simulink model "NanoBalancerCascade"  (R2022b)
settings: Solver=FixedStepAuto  StartTime=0.0  StopTime=inf  RelTol=1e-3  EnableMultiTasking=on
model workspace (MAT data in the model file):
  Saturation = 0.85
  sampleTime = 0.01
libraries: arduinomotorcarrierlib x5, simulink_extras x3, slpidlib x2, simulink x2, eeGeneralControl x2, arduinosensorlib x1, arduinolib x1
settings Model: ExtModeTrigDuration=2  Creator=arkad  LastModifiedBy=arkad
settings OptimizationCC: EnhancedBackFolding=on  PassReuseOutputArgsAs=Individual arguments  ZeroExternalMemoryAtStartup=off  ZeroInternalMemoryAtStartup=off  MaxStackSize=64  OptimizeBlockOrder=speed  DifferentSizesBufferReuse=on  OptimizationCustomize=off  EfficientTunableParamExpr=on
settings DebuggingCC: ParameterTunabilityLossMsg=error
settings HardwareCC: ProdBitPerPointer=32  ProdBitPerSizeT=32  ProdBitPerPtrDiffT=32  ProdLargestAtomicInteger=Long  ProdLargestAtomicFloat=Double  ProdWordSize=32  ProdHWDeviceType=ARM Compatible->ARM Cortex
settings SFSimCC: MATLABDynamicMemAlloc=off
settings RTWCC: Description=Embedded Coder  SystemTargetFile=ert.tlc  HardwareBoard=Arduino Nano 33 IoT  TLCOptions=-aInlineSetEventsForThisBaseRateFcn=TLC_FALSE -aSuppressMultiTaskScheduler=TLC_FALSE -aRateBasedStepFcn=1  TemplateMakefile=ert_default_tmf  Toolchain=Arduino ARM  BuildConfiguration=Faster Runs
settings CodeAppCC: ForceParamTrailComments=on  IgnoreCustomStorageClasses=off  OperatorAnnotations=on  SimulinkDataObjDesc=on  SFDataObjDesc=on  InsertBlockDesc=on
settings ERTTargetCC: SupportContinuousTime=on  SupportVariableSizeSignals=on  ExtModeTransport=2  ExtModeStaticAlloc=on  ExtModeAutomaticAllocSize=off  ExtModeStaticAllocSize=8192  ExtModeMexFile=ext_xcp  ExtModeIntrfLevel=Level2 - Open

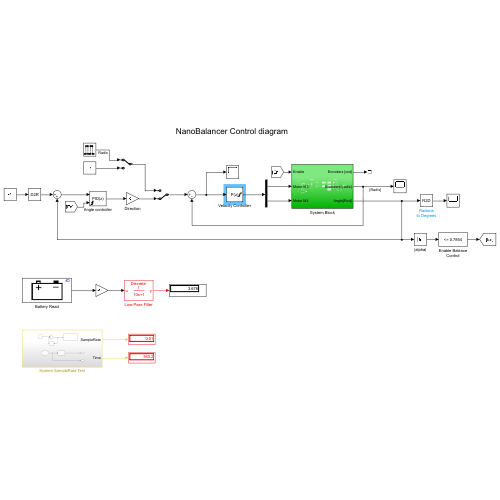
[thumbnail: Simulink's stored preview of the top-level diagram]
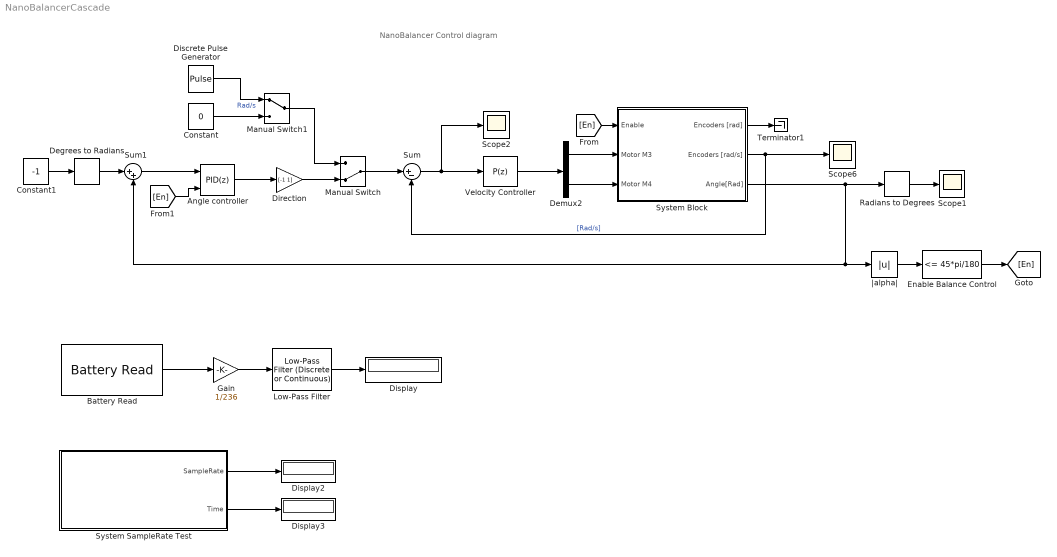
== system NanoBalancerCascade ==
  note: NanoBalancer Control diagram
  Angle controller : slpidlib/PID Controller  Controller=PID  Form=Parallel  TimeDomain=Discrete-time  UseExternalTs=off  SampleTime=-1  IntegratorMethod=Forward Euler  FilterMethod=Forward Euler  ControllerParametersSource=internal  P=175  I=10  UseKiTs=on  D=10  N=30  UseFilter=on  TunerSelectOption=Transfer Function Based (PID Tuner App)  InitialConditionSource=internal  InitialConditionForIntegrator=0  InitialConditionForFilter=0  DifferentiatorICPrevScaledInput=0  ExternalReset=rising  TrackingMode=off  Kt=1  LimitOutput=off  SatLimitsSource=internal  UpperSaturationLimit=100  LowerSaturationLimit=-100  LinearizeAsGain=on  AntiWindupMode=clamping  Kb=1  LimitIntegrator=on  UpperIntegratorSaturationLimit=50  LowerIntegratorSaturationLimit=-50  POutMin=[]  POutMax=[]  IOutMin=[]  IOutMax=[]  DOutMin=[]  DOutMax=[]  NOutMin=[]  NOutMax=[]  SumOutMin=[]  SumOutMax=[]  SaturationOutMin=[]  SaturationOutMax=[]  PParamMin=[]  PParamMax=[]  IParamMin=[]  IParamMax=[]  DParamMin=[]  DParamMax=[]  NParamMin=[]  NParamMax=[]  KbParamMin=[]  KbParamMax=[]  KtParamMin=[]  KtParamMax=[]  KbOutMin=[]  KbOutMax=[]  KtOutMin=[]  KtOutMax=[]  IntegratorOutMin=[]  IntegratorOutMax=[]  FilterOutMin=[]  FilterOutMax=[]  SumI1OutMin=[]  SumI1OutMax=[]  SumI2OutMin=[]  SumI2OutMax=[]  SumI3OutMin=[]  SumI3OutMax=[]  SumI4OutMin=[]  SumI4OutMax=[]  SumDOutMin=[]  SumDOutMax=[]  DifferentiatorOutMin=[]  DifferentiatorOutMax=[]  FilterDiffOutCoefMin=[]  FilterDiffOutCoefMax=[]  ReciprocalOutMin=[]  ReciprocalOutMax=[]  SumDenOutMin=[]  SumDenOutMax=[]  SumNumOutMin=[]  SumNumOutMax=[]  DivideOutMin=[]  DivideOutMax=[]  UdiffTsProdOutMin=[]  UdiffTsProdOutMax=[]  NTsProdOutMin=[]  NTsProdOutMax=[]  UintegralTsProdOutMin=[]  UintegralTsProdOutMax=[]  UngainTsProdOutMin=[]  UngainTsProdOutMax=[]  ClampingZeroOutDataTypeStr=Inherit: Inherit via back propagation  ClampingZeroOutMin=[]  ClampingZeroOutMax=[]  FilterDenConstantOutDataTypeStr=Inherit: Inherit via back propagation  FilterDenConstantOutMin=[]  FilterDenConstantOutMax=[]  PCopyOutDataTypeStr=Inherit: Inherit via back propagation  PCopyOutMin=[]  PCopyOutMax=[]  NCopyOutDataTypeStr=Inherit: Inherit via back propagation  NCopyOutMin=[]  NCopyOutMax=[]  IntegratorContinuousStateAttributes=''  IntegratorStateMustResolveToSignalObject=off  IntegratorRTWStateStorageClass=Auto  FilterContinuousStateAttributes=''  FilterStateMustResolveToSignalObject=off  FilterRTWStateStorageClass=Auto  ParallelPVariant=InternalParameters  IdealPVariant=Disabled  IVariant=InternalParameters  DVariant=InternalParameters  IntegratorVariant=Discrete  SatVariant=Disabled  AWVariant=Passthrough  PCopyVariant=Disabled  TRVariant=Disabled  FdbkBlocksVariant=Forward  IdealPFdbkVariant=Disabled  SatFdbkVariant=Disabled  DerivativeFilterVariant=ForwardEulerFilter  NVariant=InternalParameters  NCopyVariant=Disabled  FilterICVariant=InternalICsFilter  IntegratorICVariant=InternalICs  ExternalResetVariant=ExternalReset  TRSumVariant=Passthrough  SumFdbkVariant=Disabled  SumVariant=Sum_PID  TsampFilterVariant=InternalTs  TsampNgainVariant=Passthrough  TsampIntegralVariant=Passthrough  ExternalSaturationOutDataTypeStr=Inherit: Same as second input
  Battery Read : arduinomotorcarrierlib/Battery Read  SlaveAddress=uint8( hex2dec( '66' ) )  blockPlatform=ARDUINO  SampleTime=0.1
  Constant : Constant  Value=0
  Constant1 : Constant  Value=-1
  Degrees to Radians : simulink_extras/Transformations/Degrees to Radians
  Demux2 : Demux  Outputs=2
  Direction : Gain  Gain=[-1 1]  ParamDataTypeStr=double  OutDataTypeStr=double
  Discrete Pulse Generator : DiscretePulseGenerator  Amplitude=40  Period=4/sampleTime  PulseWidth=2/sampleTime  SampleTime=sampleTime
  Display : Display
  Display2 : Display
  Display3 : Display
  Enable Balance Control : simulink/Logic and Bit Operations/Compare To Constant  relop=<=  const=45*pi/180  OutDataTypeStr=uint8  ZeroCross=off
  Gain : Gain  Gain=1/236  ParamDataTypeStr=double  OutDataTypeStr=double
  Low-Pass Filter : eeGeneralControl/Low-Pass Filter (Discrete or Continuous)  K=1  T=10  B=inf  A=-inf  init_option=Inherited from block input  x0=0  Ts=-1
  Manual Switch : ManualSwitch  CurrentSetting=0
  Manual Switch1 : ManualSwitch
  Radians to Degrees : simulink_extras/Transformations/Radians to Degrees
  Scope1 : Scope
  Scope2 : Scope
  Scope6 : Scope
  Sum : Sum  Inputs=|+-
  Sum1 : Sum  Inputs=|++
  System Block : Subsystem
  System SampleRate Test : Subsystem
  Terminator1 : Terminator
  Velocity Controller : slpidlib/PID Controller  Controller=P  Form=Parallel  TimeDomain=Discrete-time  UseExternalTs=off  SampleTime=-1  IntegratorMethod=Forward Euler  FilterMethod=Forward Euler  ControllerParametersSource=internal  P=0.01  I=0.001*0  UseKiTs=on  D=0.01  N=20  UseFilter=on  TunerSelectOption=Transfer Function Based (PID Tuner App)  InitialConditionSource=internal  InitialConditionForIntegrator=0  InitialConditionForFilter=0  DifferentiatorICPrevScaledInput=0  ExternalReset=rising  TrackingMode=off  Kt=1  LimitOutput=on  SatLimitsSource=internal  UpperSaturationLimit=1  LowerSaturationLimit=-1  LinearizeAsGain=on  AntiWindupMode=clamping  Kb=1  LimitIntegrator=off  UpperIntegratorSaturationLimit=inf  LowerIntegratorSaturationLimit=-inf  POutMin=[]  POutMax=[]  IOutMin=[]  IOutMax=[]  DOutMin=[]  DOutMax=[]  NOutMin=[]  NOutMax=[]  SumOutMin=[]  SumOutMax=[]  SaturationOutMin=[]  SaturationOutMax=[]  PParamMin=[]  PParamMax=[]  IParamMin=[]  IParamMax=[]  DParamMin=[]  DParamMax=[]  NParamMin=[]  NParamMax=[]  KbParamMin=[]  KbParamMax=[]  KtParamMin=[]  KtParamMax=[]  KbOutMin=[]  KbOutMax=[]  KtOutMin=[]  KtOutMax=[]  IntegratorOutMin=[]  IntegratorOutMax=[]  FilterOutMin=[]  FilterOutMax=[]  SumI1OutMin=[]  SumI1OutMax=[]  SumI2OutMin=[]  SumI2OutMax=[]  SumI3OutMin=[]  SumI3OutMax=[]  SumI4OutMin=[]  SumI4OutMax=[]  SumDOutMin=[]  SumDOutMax=[]  DifferentiatorOutMin=[]  DifferentiatorOutMax=[]  FilterDiffOutCoefMin=[]  FilterDiffOutCoefMax=[]  ReciprocalOutMin=[]  ReciprocalOutMax=[]  SumDenOutMin=[]  SumDenOutMax=[]  SumNumOutMin=[]  SumNumOutMax=[]  DivideOutMin=[]  DivideOutMax=[]  UdiffTsProdOutMin=[]  UdiffTsProdOutMax=[]  NTsProdOutMin=[]  NTsProdOutMax=[]  UintegralTsProdOutMin=[]  UintegralTsProdOutMax=[]  UngainTsProdOutMin=[]  UngainTsProdOutMax=[]  ClampingZeroOutDataTypeStr=Inherit: Inherit via back propagation  ClampingZeroOutMin=[]  ClampingZeroOutMax=[]  FilterDenConstantOutDataTypeStr=Inherit: Inherit via back propagation  FilterDenConstantOutMin=[]  FilterDenConstantOutMax=[]  PCopyOutDataTypeStr=Inherit: Inherit via back propagation  PCopyOutMin=[]  PCopyOutMax=[]  NCopyOutDataTypeStr=Inherit: Inherit via back propagation  NCopyOutMin=[]  NCopyOutMax=[]  IntegratorContinuousStateAttributes=''  IntegratorStateMustResolveToSignalObject=off  IntegratorRTWStateStorageClass=Auto  FilterContinuousStateAttributes=''  FilterStateMustResolveToSignalObject=off  FilterRTWStateStorageClass=Auto  ParallelPVariant=InternalParameters  IdealPVariant=Disabled  IVariant=Disabled  DVariant=Disabled  IntegratorVariant=Disabled  SatVariant=Enabled  AWVariant=Disabled  PCopyVariant=Disabled  TRVariant=Disabled  FdbkBlocksVariant=Forward  IdealPFdbkVariant=Disabled  SatFdbkVariant=Disabled  DerivativeFilterVariant=Disabled  NVariant=Disabled  NCopyVariant=Disabled_SignalSpec  FilterICVariant=Disabled  IntegratorICVariant=Disabled  ExternalResetVariant=Disabled  TRSumVariant=Passthrough  SumFdbkVariant=Disabled  SumVariant=Passthrough_P  TsampFilterVariant=InternalTs  TsampNgainVariant=Passthrough  TsampIntegralVariant=Disabled_SignalSpec  ExternalSaturationOutDataTypeStr=Inherit: Same as second input
  |alpha| : Abs  SaturateOnIntegerOverflow=off
  wires:
  Battery Read/1 -> Gain/1
  Gain/1 -> Low-Pass Filter/1
  Low-Pass Filter/1 -> Display/1
  |alpha|/1 -> Enable Balance Control/1
  System SampleRate Test/1(SampleRate) -> Display2/1
  System SampleRate Test/2(Time) -> Display3/1
  Enable Balance Control/1 -> [En]
  Angle controller/1 -> Direction/1
  Sum1/1 -> Angle controller/1
  System Block/2(Encoders [rad/s]) -> Sum/2, Scope6/1  "[Rad/s]"
  Velocity Controller/1 -> Demux2/1
  Demux2/1 -> System Block/2(Motor M3)
  Demux2/2 -> System Block/3(Motor M4)
  Sum/1 -> Scope2/1, Velocity Controller/1
  Manual Switch/1 -> Sum/1
  System Block/3(Angle[Rad]) -> Sum1/2, |alpha|/1, Radians to Degrees/1
  [En] -> System Block/1(Enable)
  [En] -> Angle controller/2
  Constant1/1 -> Degrees to Radians/1
  System Block/1(Encoders [rad]) -> Terminator1/1
  Degrees to Radians/1 -> Sum1/1
  Radians to Degrees/1 -> Scope1/1
  Constant/1 -> Manual Switch1/2
  Manual Switch1/1 -> Manual Switch/1
  Discrete Pulse Generator/1 -> Manual Switch1/1  "Rad/s"
  Direction/1 -> Manual Switch/2

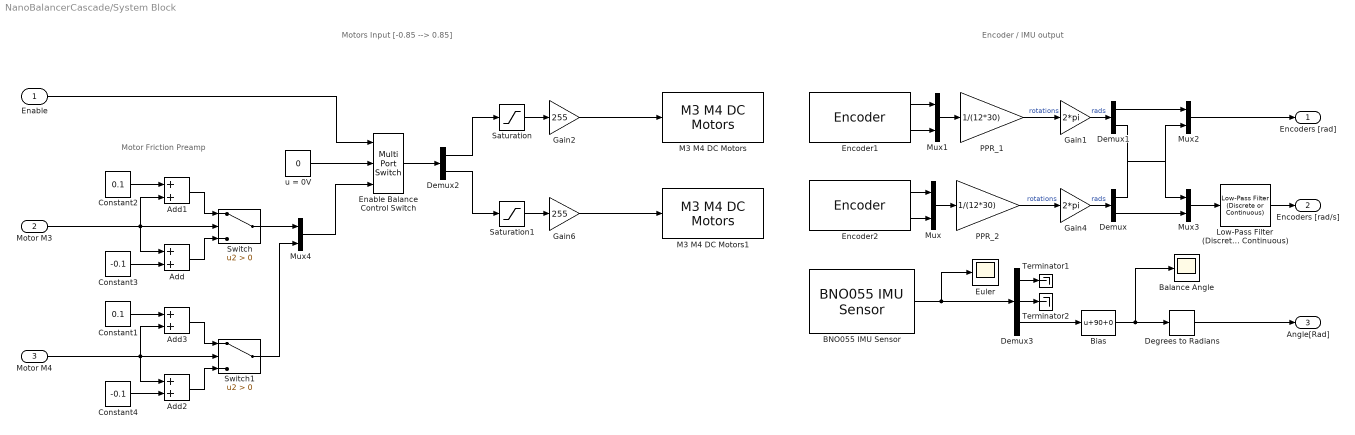
== system NanoBalancerCascade/System Block ==
  note: Motors Input [-0.85 --> 0.85]
  note: Encoder / IMU output
  note: Motor Friction Preamp
  Enable : Inport
  Motor M3 : Inport  Port=2
  Motor M4 : Inport  Port=3
  Add{,1..3} (4 alike) : Sum
  BNO055 IMU Sensor : arduinosensorlib/BNO055 IMU Sensor  SlaveAddress=0x28  OperationMode=Fusion  Accel=off  AngularRate=off  MagField=off  EulerAngles=on  Quat=off  LinearAccel=off  GravityVector=off  Status=off  Timestamp=off  AccelRange=4G  AccelBW=62.5 Hz  GyroRange=2000 dps  GyroBW=32 Hz  MagODR=10 Hz  spf=1  SampleTime=0.01  blockPlatform=ARDUINO  QueueSizeFactor=1
  Balance Angle : Scope
  Bias : Bias  Bias=90+0  SaturateOnIntegerOverflow=off
  Constant1 : Constant  Value=0.1  SampleTime=sampleTime
  Constant2 : Constant  Value=0.1  SampleTime=sampleTime
  Constant3 : Constant  Value=-0.1  SampleTime=sampleTime
  Constant4 : Constant  Value=-0.1  SampleTime=sampleTime
  Degrees to Radians : simulink_extras/Transformations/Degrees to Radians
  Demux : Demux  Outputs=2
  Demux1 : Demux  Outputs=2
  Demux2 : Demux  Outputs=2
  Demux3 : Demux  Outputs=3
  Enable Balance Control Switch : MultiPortSwitch  DataPortOrder=Zero-based contiguous  Inputs=2  zeroidx=on  SaturateOnIntegerOverflow=off  InputSameDT=off
  Encoder1 : arduinomotorcarrierlib/Encoder  SlaveAddress=uint8( hex2dec( '66' ) )  blockPlatform=ARDUINO  Encoder=1  ShowSpeed=on  ResetOption=on  SampleTime=sampleTime
  Encoder2 : arduinomotorcarrierlib/Encoder  SlaveAddress=uint8( hex2dec( '66' ) )  blockPlatform=ARDUINO  Encoder=2  ShowSpeed=on  ResetOption=on  SampleTime=sampleTime
  Euler : Scope
  Gain1 : Gain  Gain=2*pi
  Gain2 : Gain  Gain=255
  Gain4 : Gain  Gain=2*pi
  Gain6 : Gain  Gain=255
  Low-Pass Filter (Discrete or Continuous) : eeGeneralControl/Low-Pass Filter (Discrete or Continuous)  K=1  T=0.05  B=inf  A=-inf  init_option=Inherited from block input  x0=0  Ts=sampleTime
  M3 M4 DC Motors : arduinomotorcarrierlib/M3 M4 DC Motors  MotorNumber=M3  forwardPinNumber=3  reversePinNumber=2
  M3 M4 DC Motors1 : arduinomotorcarrierlib/M3 M4 DC Motors  MotorNumber=M4  forwardPinNumber=4  reversePinNumber=5
  Mux{,1..4} (5 alike) : Mux  Inputs=2
  PPR_1 : Gain  Gain=1/(12*30)  ParamDataTypeStr=double  OutDataTypeStr=double
  PPR_2 : Gain  Gain=1/(12*30)  ParamDataTypeStr=double  OutDataTypeStr=double
  Saturation : Saturate  UpperLimit=Saturation  LowerLimit=-Saturation
  Saturation1 : Saturate  UpperLimit=Saturation  LowerLimit=-Saturation
  Switch : Switch  Criteria=u2 > Threshold  SaturateOnIntegerOverflow=off  InputSameDT=off
  Switch1 : Switch  Criteria=u2 > Threshold  SaturateOnIntegerOverflow=off  InputSameDT=off
  Terminator1 : Terminator
  Terminator2 : Terminator
  u = 0V : Constant  Value=0
  Encoders [rad] : Outport
  Encoders [rad/s] : Outport  Port=2
  Angle[Rad] : Outport  Port=3
  wires:
  Gain2/1 -> M3 M4 DC Motors/1
  Saturation/1 -> Gain2/1
  Saturation1/1 -> Gain6/1
  Gain6/1 -> M3 M4 DC Motors1/1
  PPR_2/1 -> Gain4/1  "rotations"
  PPR_1/1 -> Gain1/1  "rotations"
  Encoder2/1 -> Mux/1
  Encoder2/2 -> Mux/2
  Mux/1 -> PPR_2/1
  Mux1/1 -> PPR_1/1
  Encoder1/1 -> Mux1/1
  Encoder1/2 -> Mux1/2
  Gain4/1 -> Demux/1  "rads"
  Gain1/1 -> Demux1/1  "rads"
  Demux1/1 -> Mux2/1
  Demux1/2 -> Mux3/1
  Demux/1 -> Mux2/2
  Demux/2 -> Mux3/2
  Mux2/1 -> Encoders [rad]/1
  Mux3/1 -> Low-Pass Filter (Discrete or Continuous)/1
  Enable/1 -> Enable Balance Control Switch/1
  u = 0V/1 -> Enable Balance Control Switch/2
  Enable Balance Control Switch/1 -> Demux2/1
  Demux2/1 -> Saturation/1
  Demux2/2 -> Saturation1/1
  Add1/1 -> Switch/1
  Constant3/1 -> Add/2
  Add/1 -> Switch/3
  Constant2/1 -> Add1/1
  Motor M3/1 -> Add1/2, Add/1, Switch/2
  Demux3/3 -> Bias/1
  Demux3/1 -> Terminator1/1
  Demux3/2 -> Terminator2/1
  BNO055 IMU Sensor/1 -> Demux3/1, Euler/1
  Bias/1 -> Balance Angle/1, Degrees to Radians/1
  Degrees to Radians/1 -> Angle[Rad]/1
  Mux4/1 -> Enable Balance Control Switch/3
  Motor M4/1 -> Add3/2, Add2/1, Switch1/2
  Add2/1 -> Switch1/3
  Constant4/1 -> Add2/2
  Add3/1 -> Switch1/1
  Constant1/1 -> Add3/1
  Switch1/1 -> Mux4/2
  Switch/1 -> Mux4/1
  Low-Pass Filter (Discrete or Continuous)/1 -> Encoders [rad/s]/1

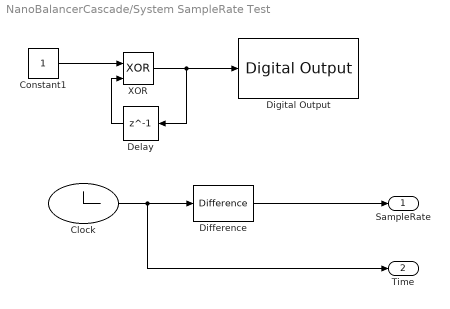
== system NanoBalancerCascade/System SampleRate Test ==
  Clock : Clock
      settings: Decimation=3
  Constant1 : Constant  SampleTime=sampleTime
  Delay : Delay  DelayLength=1  InitialCondition=0  SampleTime=sampleTime
  Difference : simulink/Quick Insert/Discrete/Difference  ICPrevInput=0.0  OutMin=[]  OutMax=[]  OutDataType=fixdt(1, 16)  OutScaling=2^-10  DoSatur=off
  Digital Output : arduinolib/Digital Output  pinNumber=13  Direction=output  blockPlatform=arduino
  XOR : Logic  Operator=XOR  IconShape=distinctive  AllPortsSameDT=off  OutDataTypeStr=boolean
  SampleRate : Outport
  Time : Outport  Port=2
  wires:
  XOR/1 -> Delay/1, Digital Output/1
  Constant1/1 -> XOR/1
  Delay/1 -> XOR/2
  Clock/1 -> Time/1, Difference/1
  Difference/1 -> SampleRate/1
